simulink model "ABS_example_model"  (R2023b)
settings: Solver=VariableStepAuto  StartTime=0.0  StopTime=10.0  RelTol=1e-3
settings Model: Creator=Santhosh  LastModifiedBy=Santhosh

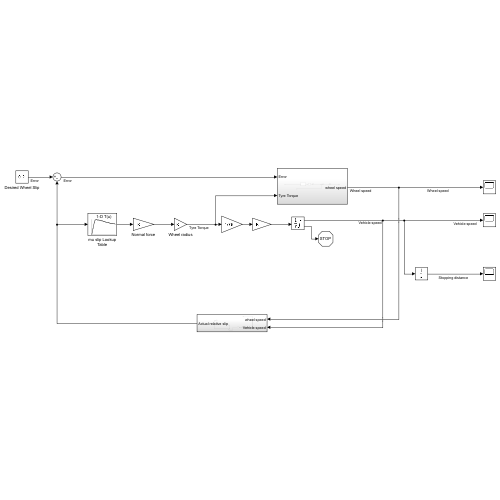
[thumbnail: Simulink's stored preview of the top-level diagram]
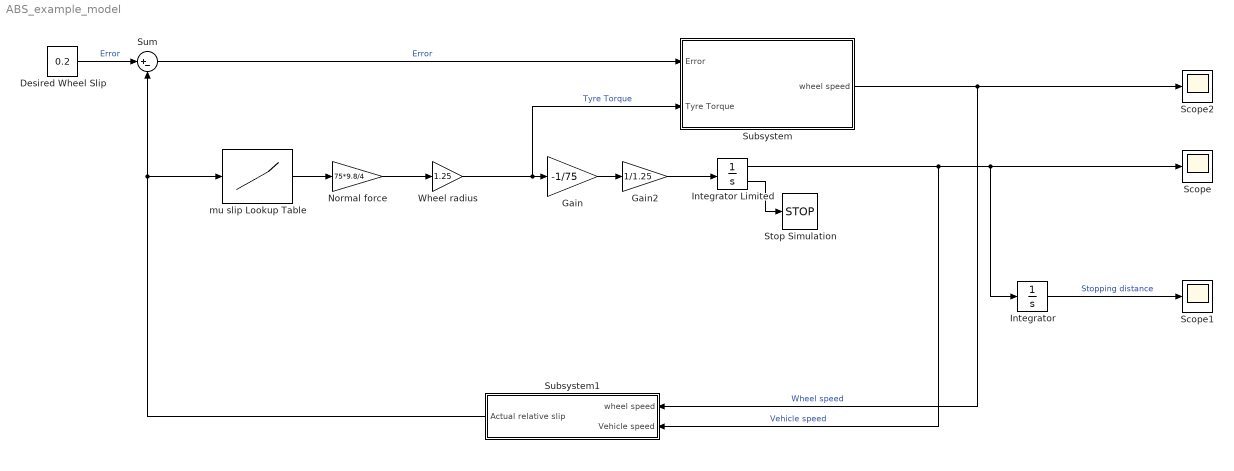
== system ABS_example_model ==
  Desired Wheel Slip : Constant  Value=0.2
  Gain : Gain  Gain=-1/75
  Gain2 : Gain  Gain=1/1.25
  Integrator : Integrator
  Integrator Limited : Integrator  InitialCondition=44  LimitOutput=on  UpperSaturationLimit=2000  LowerSaturationLimit=0  ShowSaturationPort=on
  Normal force : Gain  Gain=75*9.8/4
  Scope : Scope
  Scope1 : Scope
  Scope2 : Scope
  Stop Simulation : Stop
  Subsystem : Subsystem
  Subsystem1 : Subsystem
  Sum : Sum  Inputs=|+-
  Wheel radius : Gain  Gain=1.25
  mu slip Lookup Table : Lookup_n-D  NumberOfTableDimensions=1  BreakpointsForDimension1=[0;0.05;0.1;0.15;0.2;0.25;0.3;0.35;0.4;0.45;0.5;0.55;0.6;0.65;0.7;0.75;0.8;0.85;0.9;0.95;1]  Table=[0;0.4;0.8;0.97;1;0.98;0.96;0.94;0.92;0.9;0.88;0.855;0.83;0.81;0.79;0.77;0.75;0.73;0.72;0.71;0.7]  InternalRulePriority=Speed  RndMeth=Simplest
  wires:
  Desired Wheel Slip/1 -> Sum/1  "Error"
  mu slip Lookup Table/1 -> Normal force/1
  Normal force/1 -> Wheel radius/1
  Sum/1 -> Subsystem/1(Error)  "Error"
  Wheel radius/1 -> Gain/1, Subsystem/2(Tyre Torque)  "Tyre Torque"
  Gain/1 -> Gain2/1
  Integrator Limited/1 -> Subsystem1/2(Vehicle speed), Integrator/1, Scope/1  "Vehicle speed"
  Integrator/1 -> Scope1/1  "Stopping distance"
  Subsystem1/1(Actual relative slip) -> mu slip Lookup Table/1, Sum/2
  Subsystem/1(wheel speed) -> Subsystem1/1(wheel speed), Scope2/1  "Wheel speed"
  Gain2/1 -> Integrator Limited/1
  Integrator Limited/2 -> Stop Simulation/1

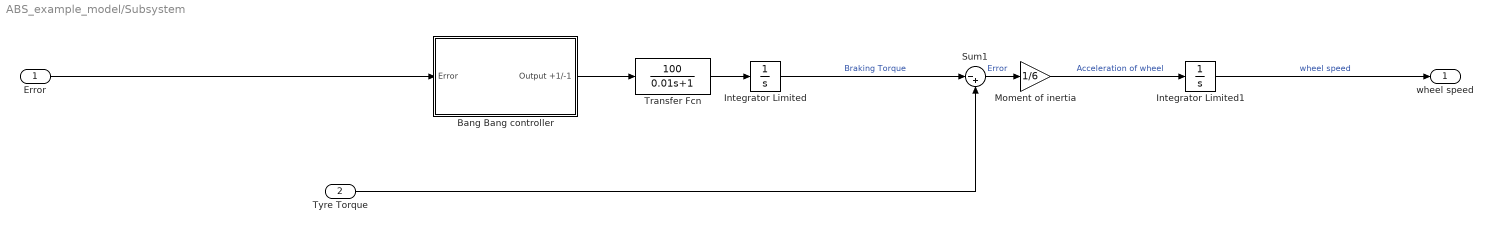
== system ABS_example_model/Subsystem ==
  Error : Inport
  Tyre Torque : Inport  Port=2
  Bang Bang controller : Subsystem
  Integrator Limited : Integrator  InitialCondition=44/1.25  LimitOutput=on  UpperSaturationLimit=2000  LowerSaturationLimit=0
  Integrator Limited1 : Integrator  InitialCondition=44  LimitOutput=on  UpperSaturationLimit=1000  LowerSaturationLimit=0
  Moment of inertia : Gain  Gain=1/6
  Sum1 : Sum  Inputs=|-+
  Transfer Fcn : TransferFcn  Numerator=[100]  Denominator=[0.01 1]
  wheel speed : Outport
  wires:
  Integrator Limited/1 -> Sum1/1  "Braking Torque"
  Bang Bang controller/1(Output +1/-1) -> Transfer Fcn/1
  Integrator Limited1/1 -> wheel speed/1  "wheel speed"
  Moment of inertia/1 -> Integrator Limited1/1  "Acceleration of wheel"
  Transfer Fcn/1 -> Integrator Limited/1
  Sum1/1 -> Moment of inertia/1  "Error"
  Tyre Torque/1 -> Sum1/2
  Error/1 -> Bang Bang controller/1(Error)

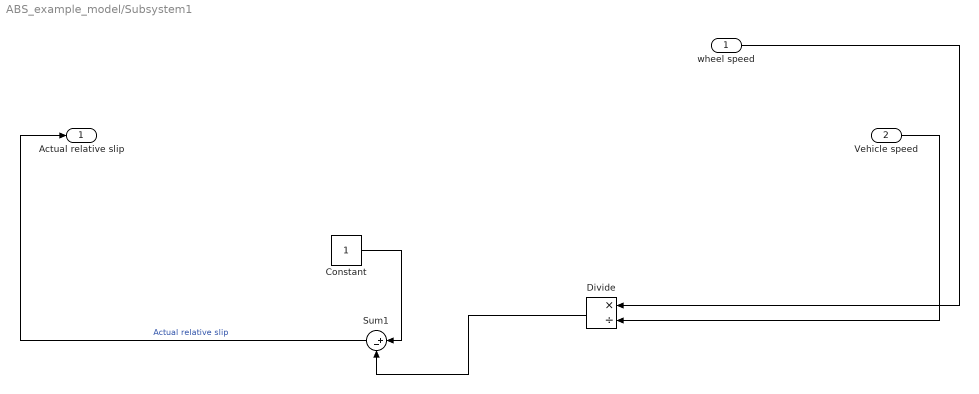
== system ABS_example_model/Subsystem1 ==
  wheel speed : Inport
  Vehicle speed : Inport  Port=2
  Constant : Constant
  Divide : Product  Inputs=*/
  Sum1 : Sum  Inputs=|+-
  Actual relative slip : Outport
  wires:
  Constant/1 -> Sum1/1
  Vehicle speed/1 -> Divide/2
  Divide/1 -> Sum1/2
  Sum1/1 -> Actual relative slip/1  "Actual relative slip"
  wheel speed/1 -> Divide/1

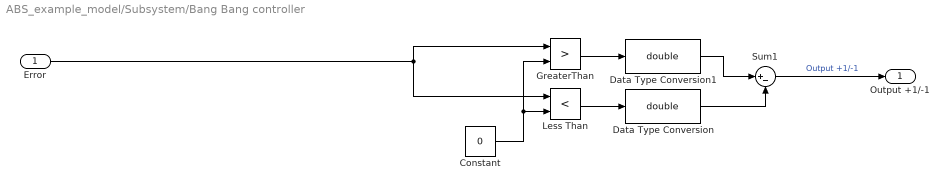
== system ABS_example_model/Subsystem/Bang Bang controller ==
  Error : Inport
  Constant : Constant  Value=0
  Data Type Conversion : DataTypeConversion  OutDataTypeStr=double  SaturateOnIntegerOverflow=off
  Data Type Conversion1 : DataTypeConversion  OutDataTypeStr=double  SaturateOnIntegerOverflow=off
  GreaterThan : RelationalOperator  Operator=>  OutDataTypeStr=boolean  RndMeth=Simplest  InputSameDT=off
  Less Than : RelationalOperator  Operator=<  OutDataTypeStr=boolean  RndMeth=Simplest  InputSameDT=off
  Sum1 : Sum  Inputs=|+-
  Output +1/-1 : Outport
  wires:
  Data Type Conversion/1 -> Sum1/2
  Constant/1 -> GreaterThan/2, Less Than/2
  Less Than/1 -> Data Type Conversion/1
  Data Type Conversion1/1 -> Sum1/1
  GreaterThan/1 -> Data Type Conversion1/1
  Error/1 -> GreaterThan/1, Less Than/1
  Sum1/1 -> Output +1/-1/1  "Output +1/-1"
